simulink model "OBSTACLE_DETECTION_FINAL"  (R2020a)
settings: Solver=ode3  StartTime=0.0  StopTime=inf  FixedStep=0.01  RelTol=1e-3  EnableMultiTasking=on
libraries: robotlib x9
Description:
  | Software-in-the-Loop Code Verification
settings Model: ModifiedByFormat=The MathWorks Inc.  ExtModeTrigDuration=2  ExtModeAutoUpdateStatusClock=off  Creator=The MathWorks, Inc.  LastModifiedBy=The MathWorks Inc.
settings SolverCC: PositivePriorityOrder=on
settings DataIOCC: SaveFormat=Array  SignalLogging=off  SignalLoggingName=sigsOut
settings OptimizationCC: UseDivisionForNetSlopeComputation=UseDivisionForReciprocalsOfIntegersOnly  EnhancedBackFolding=on  BooleansAsBitfields=on  PassReuseOutputArgsAs=Individual arguments  ExpressionDepthLimit=2147483647  StateBitsets=on  DataBitsets=on  ZeroExternalMemoryAtStartup=off  ZeroInternalMemoryAtStartup=off  NoFixptDivByZeroProtection=on  EfficientFloat2IntCast=on  LifeSpan=1  MaxStackSize=64  EfficientTunableParamExpr=on
settings DebuggingCC: CheckExecutionContextPreStartOutputMsg=on  CheckExecutionContextRuntimeOutputMsg=on  FcnCallInpInsideContextMsg=warning  UnconnectedLineMsg=none  AllowSymbolicDim=off  StateNameClashWarn=warning  StrictBusMsg=ErrorOnBusTreatedAsVector  SymbolicDimsDataTypeCodeGenerationDiagnostic=none  SFUnexpectedBacktrackingDiag=warning  SFNoUnconditionalDefaultTransitionDiag=warning  SFExecutionAtInitializationDiag=none  ArithmeticOperatorsInVariantConditions=warning
settings HardwareCC: ProdBitPerInt=16  ProdBitPerPointer=16  ProdBitPerSizeT=16  ProdBitPerPtrDiffT=16  ProdLargestAtomicFloat=None  ProdWordSize=8  ProdHWDeviceType=Atmel->AVR  TargetBitPerLong=64  TargetBitPerPointer=64  TargetBitPerSizeT=64  TargetBitPerPtrDiffT=64  TargetLongLongMode=on  TargetIntDivRoundTo=Zero  TargetEndianess=LittleEndian  TargetWordSize=64  TargetHWDeviceType=Generic->MATLAB Host Computer
settings ModelReferenceCC: PropagateSignalLabelsOutOfModel=off
settings SFSimCC: SimUseLocalCustomCode=off  MATLABDynamicMemAlloc=off
settings RTWCC: SystemTargetFile=ert.tlc  HardwareBoard=Arduino Mega 2560  TemplateMakefile=ert_default_tmf  GenerateReport=on  RTWVerbose=off  RTWUseLocalCustomCode=off  Toolchain=Arduino AVR  BuildConfiguration=Faster Runs  IncludeHyperlinkInReport=on  PortableWordSizes=on  CreateSILPILBlock=PIL  GenerateTraceInfo=on  GenerateTraceReport=on  GenerateTraceReportSl=on  GenerateTraceReportSf=on  GenerateTraceReportEml=on  GenerateCodeMetricsReport=on
settings CodeAppCC: ForceParamTrailComments=on  IgnoreCustomStorageClasses=off  IgnoreTestpoints=on  SimulinkDataObjDesc=on  CustomSymbolStrGlobalVar=rt$N$M  CustomSymbolStrType=$N$M  CustomSymbolStrFcn=$N$M$F  CustomSymbolStrModelFcn=$N  CustomSymbolStrMacro=$N$M  InsertBlockDesc=on  StateflowObjectComments=on  InternalIdentifier=Classic
settings ERTTargetCC: UtilityFuncGeneration=Shared location  MultiwordLength=2048  IncludeMdlTerminateFcn=off  CombineSignalStateStructs=on  SupportNonFinite=off  SupportComplex=off  SupportContinuousTime=on  SupportVariableSizeSignals=on  ERTFilePackagingFormat=CompactWithDataFile  ConvertIfToSwitch=off  SuppressUnreachableDefaultCases=off
settings ConfigComp: CovMetricSettings=dw  CovHtmlReporting=on  CovSaveCumulativeToWorkspaceVar=on  CovSaveSingleToWorkspaceVar=on  CovExternalEMLEnable=off  CovSFcnEnable=off

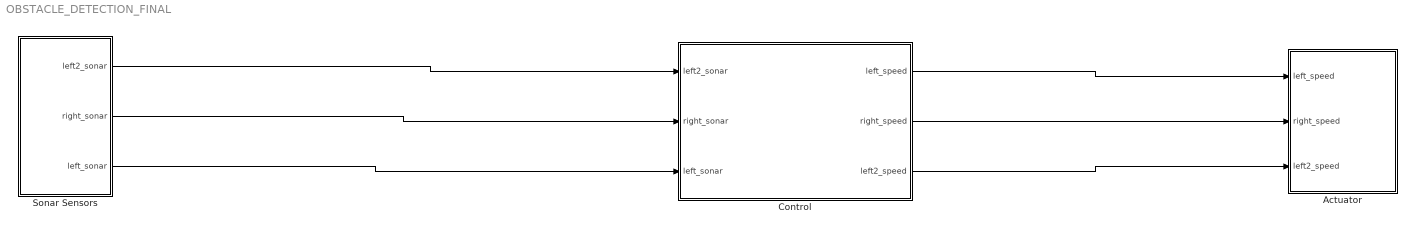
== system OBSTACLE_DETECTION_FINAL ==
  Actuator : Subsystem
  Control : Subsystem
  Sonar Sensors : Subsystem
  wires:
  Sonar Sensors/1(left2_sonar) -> Control/1(left2_sonar)
  Sonar Sensors/2(right_sonar) -> Control/2(right_sonar)
  Sonar Sensors/3(left_sonar) -> Control/3(left_sonar)
  Control/1(left_speed) -> Actuator/1(left_speed)
  Control/2(right_speed) -> Actuator/2(right_speed)
  Control/3(left2_speed) -> Actuator/3(left2_speed)

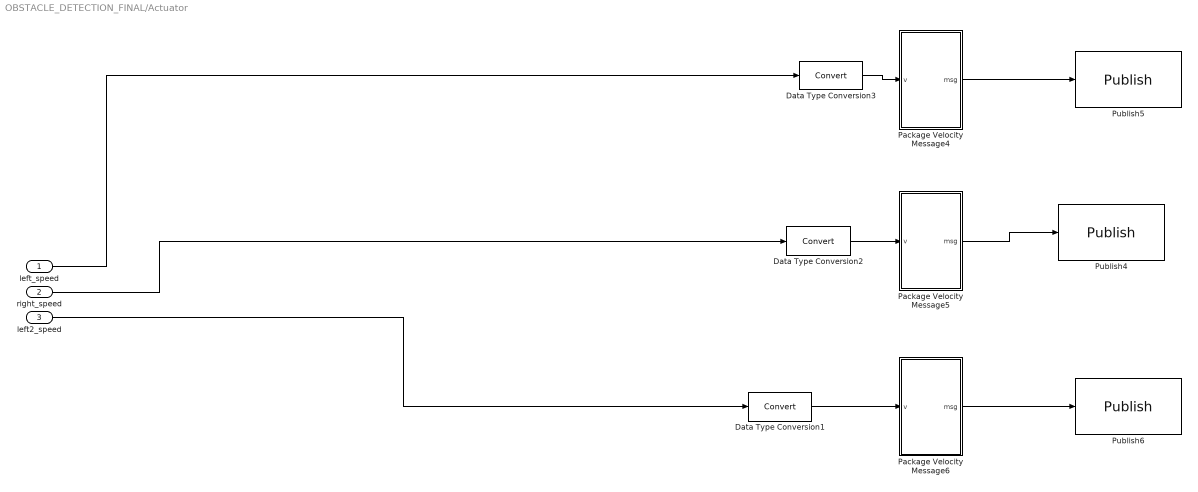
== system OBSTACLE_DETECTION_FINAL/Actuator ==
  left_speed : Inport
  right_speed : Inport  Port=2
  left2_speed : Inport  Port=3
  Data Type Conversion1 : DataTypeConversion
  Data Type Conversion2 : DataTypeConversion
  Data Type Conversion3 : DataTypeConversion
  Package Velocity Message4 : Subsystem
  Package Velocity Message5 : Subsystem
  Package Velocity Message6 : Subsystem
  Publish4 : robotlib/Publish  topicSource=Select from ROS network  topic=/robot/right_joint_velocity_controller/command  messageType=std_msgs/Float64  messageQueueLength=1
  Publish5 : robotlib/Publish  topicSource=Select from ROS network  topic=/robot/left_joint_velocity_controller/command  messageType=std_msgs/Float64  messageQueueLength=1
  Publish6 : robotlib/Publish  topicSource=Select from ROS network  topic=/robot/left2_joint_velocity_controller/command  messageType=std_msgs/Float64  messageQueueLength=1
  wires:
  left_speed/1 -> Data Type Conversion3/1
  Package Velocity Message6/1(msg) -> Publish6/1
  right_speed/1 -> Data Type Conversion2/1
  Package Velocity Message4/1(msg) -> Publish5/1
  Package Velocity Message5/1(msg) -> Publish4/1
  left2_speed/1 -> Data Type Conversion1/1
  Data Type Conversion1/1 -> Package Velocity Message6/1(v)
  Data Type Conversion2/1 -> Package Velocity Message5/1(v)
  Data Type Conversion3/1 -> Package Velocity Message4/1(v)

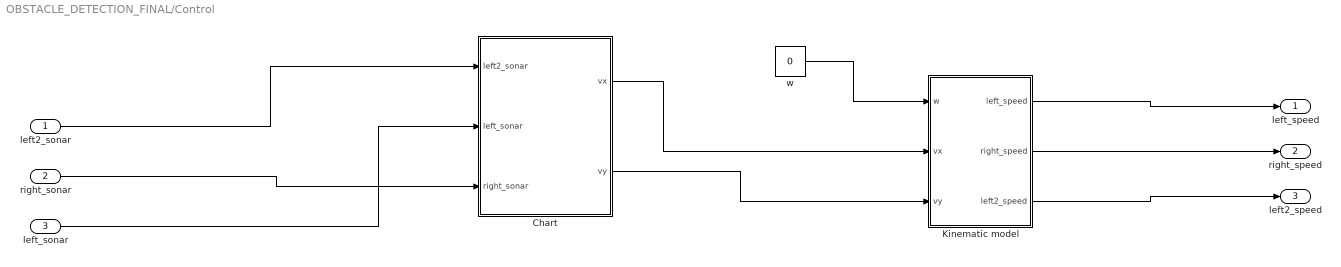
== system OBSTACLE_DETECTION_FINAL/Control ==
  left2_sonar : Inport
  right_sonar : Inport  Port=2
  left_sonar : Inport  Port=3
  Chart : Stateflow chart  TreatAsAtomicUnit=on
  Kinematic model : Subsystem
  w : Constant  Value=0  OutDataTypeStr=single
  left_speed : Outport
  right_speed : Outport  Port=2
  left2_speed : Outport  Port=3
  wires:
  left_sonar/1 -> Chart/2(left_sonar)
  w/1 -> Kinematic model/1(w)
  Kinematic model/1(left_speed) -> left_speed/1
  Chart/1(vx) -> Kinematic model/2(vx)
  Chart/2(vy) -> Kinematic model/3(vy)
  right_sonar/1 -> Chart/3(right_sonar)
  left2_sonar/1 -> Chart/1(left2_sonar)
  Kinematic model/3(left2_speed) -> left2_speed/1
  Kinematic model/2(right_speed) -> right_speed/1

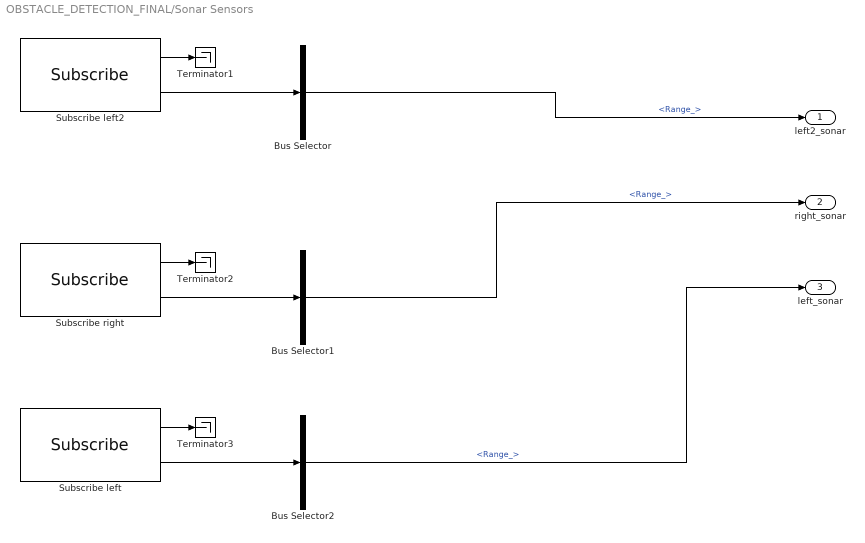
== system OBSTACLE_DETECTION_FINAL/Sonar Sensors ==
  Bus Selector : BusSelector  OutputSignals=Range_
  Bus Selector1 : BusSelector  OutputSignals=Range_
  Bus Selector2 : BusSelector  OutputSignals=Range_
  Subscribe left : robotlib/Subscribe  topicSource=Select from ROS network  topic=/sonar_sonar_link_3  messageType=sensor_msgs/Range  sampleTime=-1  messageQueueLength=1
  Subscribe left2 : robotlib/Subscribe  topicSource=Select from ROS network  topic=/sonar_sonar_link_1  messageType=sensor_msgs/Range  sampleTime=-1  messageQueueLength=1
  Subscribe right : robotlib/Subscribe  topicSource=Select from ROS network  topic=/sonar_sonar_link_2  messageType=sensor_msgs/Range  sampleTime=-1  messageQueueLength=1
  Terminator1 : Terminator
  Terminator2 : Terminator
  Terminator3 : Terminator
  left2_sonar : Outport
  right_sonar : Outport  Port=2
  left_sonar : Outport  Port=3
  wires:
  Bus Selector1/1 -> right_sonar/1  "<Range_>"
  Subscribe left/1 -> Terminator3/1
  Subscribe left/2 -> Bus Selector2/1
  Subscribe left2/1 -> Terminator1/1
  Subscribe right/1 -> Terminator2/1
  Bus Selector/1 -> left2_sonar/1  "<Range_>"
  Subscribe right/2 -> Bus Selector1/1
  Subscribe left2/2 -> Bus Selector/1
  Bus Selector2/1 -> left_sonar/1  "<Range_>"

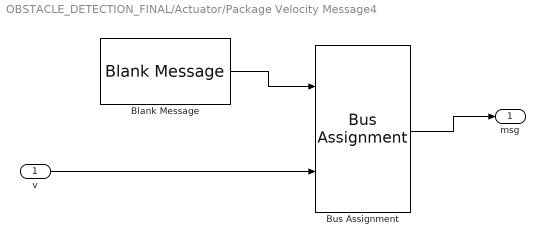
== system OBSTACLE_DETECTION_FINAL/Actuator/Package Velocity Message4 ==
  v : Inport
  Blank Message : robotlib/Blank Message  messageClass=Message  entityType=std_msgs/Float64  messageType=std_msgs/Float64  SampleTime=inf
  Bus Assignment : BusAssignment  AssignedSignals=Data
  msg : Outport  VectorParamsAs1DForOutWhenUnconnected=off
  wires:
  Blank Message/1 -> Bus Assignment/1
  Bus Assignment/1 -> msg/1
  v/1 -> Bus Assignment/2

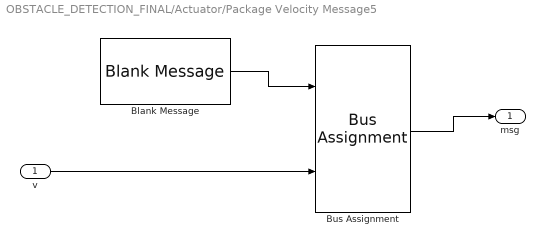
== system OBSTACLE_DETECTION_FINAL/Actuator/Package Velocity Message5 ==
  v : Inport
  Blank Message : robotlib/Blank Message  messageClass=Message  entityType=std_msgs/Float64  messageType=std_msgs/Float64  SampleTime=inf
  Bus Assignment : BusAssignment  AssignedSignals=Data
  msg : Outport  VectorParamsAs1DForOutWhenUnconnected=off
  wires:
  Blank Message/1 -> Bus Assignment/1
  Bus Assignment/1 -> msg/1
  v/1 -> Bus Assignment/2

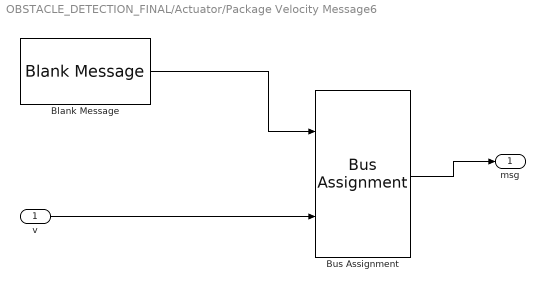
== system OBSTACLE_DETECTION_FINAL/Actuator/Package Velocity Message6 ==
  v : Inport
  Blank Message : robotlib/Blank Message  messageClass=Message  entityType=std_msgs/Float64  messageType=std_msgs/Float64  SampleTime=inf
  Bus Assignment : BusAssignment  AssignedSignals=Data
  msg : Outport  VectorParamsAs1DForOutWhenUnconnected=off
  wires:
  Blank Message/1 -> Bus Assignment/1
  Bus Assignment/1 -> msg/1
  v/1 -> Bus Assignment/2

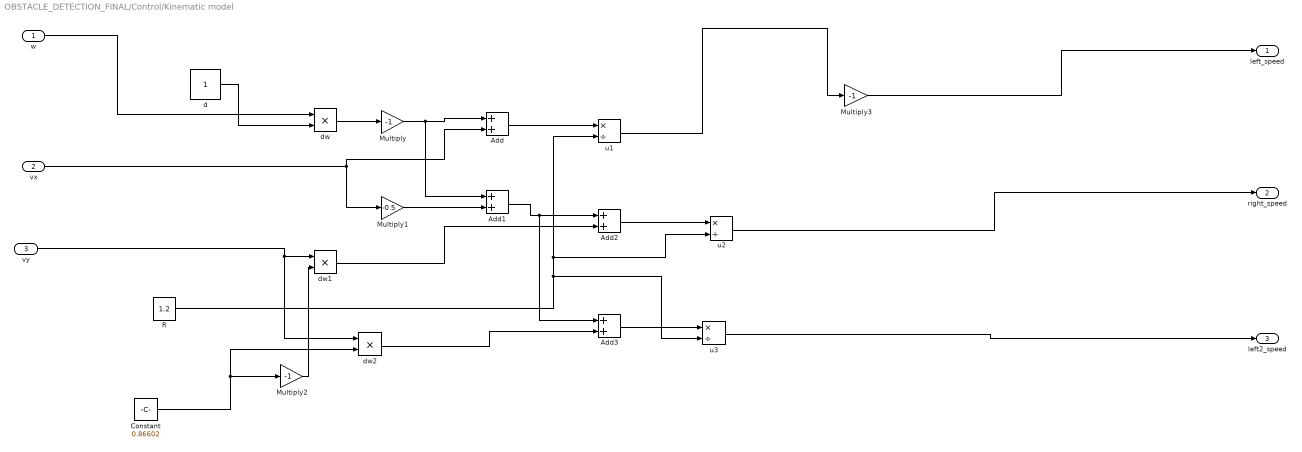
== system OBSTACLE_DETECTION_FINAL/Control/Kinematic model ==
  w : Inport  OutDataTypeStr=single
  vx : Inport  Port=2  OutDataTypeStr=single
  vy : Inport  Port=3  OutDataTypeStr=single
  Add{,1..3} (4 alike) : Sum  OutDataTypeStr=single
  Constant : Constant  Value=0.86602  OutDataTypeStr=single
  Multiply : Gain  Gain=-1  OutDataTypeStr=single
  Multiply1 : Gain  Gain=-0.5  OutDataTypeStr=single
  Multiply2 : Gain  Gain=-1  OutDataTypeStr=single
  Multiply3 : Gain  Gain=-1  OutDataTypeStr=single
  R : Constant  Value=1.2  OutDataTypeStr=single
  d : Constant  VectorParams1D=off  OutDataTypeStr=single  SampleTime=-1
  dw : Product  OutDataTypeStr=single
  dw1 : Product  OutDataTypeStr=single
  dw2 : Product  OutDataTypeStr=single
  u1 : Product  Inputs=*/  OutDataTypeStr=single
  u2 : Product  Inputs=*/  OutDataTypeStr=single
  u3 : Product  Inputs=*/  OutDataTypeStr=single
  left_speed : Outport  OutDataTypeStr=single
  right_speed : Outport  Port=2  OutDataTypeStr=single
  left2_speed : Outport  Port=3  OutDataTypeStr=single
  wires:
  Multiply/1 -> Add1/1, Add/1
  Add/1 -> u1/1
  Multiply3/1 -> left_speed/1
  dw1/1 -> Add2/2
  w/1 -> dw/1
  Multiply2/1 -> dw1/2
  Add1/1 -> Add3/1, Add2/1
  Constant/1 -> dw2/2, Multiply2/1
  u3/1 -> left2_speed/1
  vy/1 -> dw2/1, dw1/1
  dw2/1 -> Add3/2
  d/1 -> dw/2
  u2/1 -> right_speed/1
  R/1 -> u3/2, u2/2, u1/2
  Add3/1 -> u3/1
  dw/1 -> Multiply/1
  vx/1 -> Add/2, Multiply1/1
  u1/1 -> Multiply3/1
  Add2/1 -> u2/1
  Multiply1/1 -> Add1/2

== stateflow chart OBSTACLE_DETECTION_FINAL/Control/Chart ==
  state left2_obs
    entry:
    vx = speed_gain;
    vy = 0.57735026919 *speed_gain;
  state INIT
    entry:
    speed_gain = 7;
    vy = 10;
  state MAIN_STATE
  state left_left2_obs
    entry:
    vx = speed_gain;
    vy = -0.57735026919 *speed_gain;
  state left_right_obs
    entry:
    vy = -0.57735026919 * speed_gain ;
    vx = -1*speed_gain;
  state right_obs
    entry:
    vx = -1*speed_gain;
    vy = 0.57735026919 *speed_gain;
  state right_left2_obs
    entry:
    vx = 0;
    vy = speed_gain;
  state left_obs
    entry:
    vx = 0;
    vy =-1*speed_gain;
  MAIN_STATE -> left2_obs [order 1] : [left2_sonar >= 1 && left_sonar < 1 && right_sonar <1 ]
  left2_obs -> MAIN_STATE : [~(left2_sonar >= 1 && left_sonar < 1 && right_sonar <1) ]
  (default) -> INIT
  INIT -> MAIN_STATE
  MAIN_STATE -> left_right_obs [order 6] : [left2_sonar < 1 && left_sonar >= 1 && right_sonar >=1 ]
  left_left2_obs -> MAIN_STATE : [~(left2_sonar >= 1 && left_sonar >= 1 && right_sonar <1) ]
  MAIN_STATE -> left_left2_obs [order 4] : [left2_sonar >= 1 && left_sonar >= 1 && right_sonar <1 ]
  left_right_obs -> MAIN_STATE : [~(left2_sonar < 1 && left_sonar >= 1 && right_sonar >=1 )]
  right_obs -> MAIN_STATE : [~(left2_sonar < 1 && left_sonar < 1 && right_sonar >1) ]
  MAIN_STATE -> right_left2_obs [order 5] : [left2_sonar >= 1 && left_sonar < 1 && right_sonar >=1 ]
  right_left2_obs -> MAIN_STATE : [~(left2_sonar >= 1 && left_sonar < 1 && right_sonar >=1) ]
  MAIN_STATE -> right_obs [order 2] : [left2_sonar < 1 && left_sonar < 1 && right_sonar >1 ]
  MAIN_STATE -> left_obs [order 3] : [left2_sonar < 1 && left_sonar >= 1 && right_sonar <1 ]
  left_obs -> MAIN_STATE : [~(left2_sonar < 1 && left_sonar >= 1 && right_sonar <1) ]
  data: left2_sonar input single; vx output single; vy output single; speed_gain local single; left_sonar input single; right_sonar input single
